simulink model "vehicle_directDrive_Torque"  (R2015a)
settings: Solver=ode23t  StartTime=0.0  StopTime=100  RelTol=1e-3  AbsTol=1e-3
PreLoadFcn:
  | car_tire_data
values from neighbouring files (symbols this model uses):
  rider_mass = 80    [car_tire_data.m]
  tire_dia = 18    [car_tire_data.m]
  vehicle_mass = 237    [car_tire_data.m]
libraries: fl_lib x13, nesl_utility x13, sdl_lib x5
settings Model: Creator=sseshadr  LastModifiedBy=sseshadr
settings SimscapeCC: SimscapeLogType=all  SimscapeLogDataHistory=10000

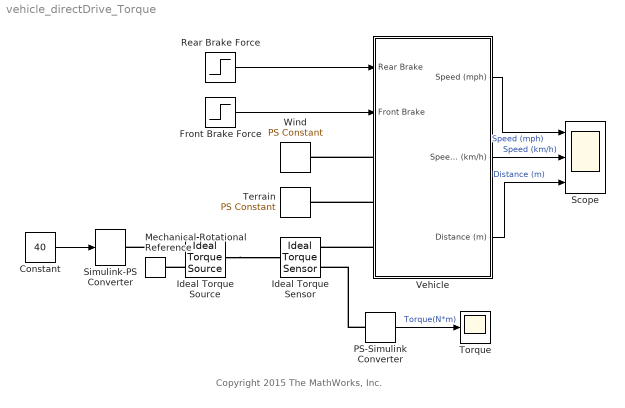
== system vehicle_directDrive_Torque ==
  note: Copyright 2015 The MathWorks, Inc.
  Constant : Constant  Value=40
  Front Brake Force : Step  Time=75  After=200  SampleTime=0
      settings: AttributesFormatString=%<After> N at %<Time> s
  Ideal Torque Sensor : fl_lib/Mechanical/Mechanical Sensors/Ideal Torque Sensor
  Ideal Torque Source : fl_lib/Mechanical/Mechanical Sources/Ideal Torque Source
  Mechanical Rotational Reference : fl_lib/Mechanical/Rotational Elements/Mechanical Rotational Reference
  PS-Simulink Converter : nesl_utility/PS-Simulink Converter  PhysicalDomain=network_engine_domain  SubClassName=ps_output  LeftPortType=input  RightPortType=output  PseudoPeriodic=off  Frequencies=[]  Unit=N*m  AffineConversion=off
  Rear Brake Force : Step  Time=50  After=100  SampleTime=0
      settings: AttributesFormatString=%<After> N at %<Time> s
  Scope : Scope  NumInputPorts=3
      settings: YMin=-5~-5~-5  YMax=5~5~5
  Simulink-PS Converter : nesl_utility/Simulink-PS Converter  PhysicalDomain=network_engine_domain  SubClassName=ps_input  LeftPortType=input  RightPortType=output  PseudoPeriodic=off  Frequencies=[]  NoiseDistribution=none  NoiseParameters=[]  Unit=N*m  AffineConversion=off  InputFiltering=off  SimscapeFilterOrder=1  InputFilterTimeConstant=0.001  UdotUserProvided=1
  Terrain : fl_lib/Physical Signals/Sources/PS Constant  constant=0
  Torque : Scope
      settings: TimeRange=40  YMin=-100  YMax=1000  SaveName=ScopeData2
  Vehicle : Subsystem
  Wind : fl_lib/Physical Signals/Sources/PS Constant  constant=0
  wires:
  Rear Brake Force/1 -> Vehicle/1(Rear Brake)
  Vehicle/1(Speed (mph)) -> Scope/1  "Speed (mph)"
  Vehicle/2(Speed (km/h)) -> Scope/2  "Speed (km/h)"
  Vehicle/3(Distance (m)) -> Scope/3  "Distance (m)"
  Front Brake Force/1 -> Vehicle/2(Front Brake)
  Constant/1 -> Simulink-PS Converter/1
  PS-Simulink Converter/1 -> Torque/1  "Torque(N*m)"
  connections:
  Vehicle/LConn1 -- Wind/RConn1
  Vehicle/LConn2 -- Terrain/RConn1
  Ideal Torque Source/RConn1 -- Simulink-PS Converter/RConn1
  Vehicle/LConn3 -- Ideal Torque Sensor/RConn1
  Ideal Torque Source/RConn2 -- Mechanical Rotational Reference/LConn1
  PS-Simulink Converter/LConn1 -- Ideal Torque Sensor/RConn2
  Ideal Torque Source/LConn1 -- Ideal Torque Sensor/LConn1

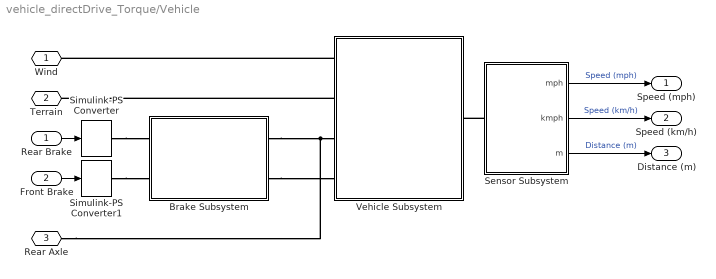
== system vehicle_directDrive_Torque/Vehicle ==
  Rear Brake : Inport
  Front Brake : Inport  Port=2
  Brake Subsystem : Subsystem
  Sensor Subsystem : Subsystem
  Simulink-PS Converter : nesl_utility/Simulink-PS Converter  PhysicalDomain=network_engine_domain  SubClassName=ps_input  LeftPortType=input  RightPortType=output  PseudoPeriodic=off  Frequencies=[]  NoiseDistribution=none  NoiseParameters=[]  Unit=1  AffineConversion=off  InputFiltering=on  SimscapeFilterOrder=1  InputFilterTimeConstant=0.001  UdotUserProvided=1
  Simulink-PS Converter1 : nesl_utility/Simulink-PS Converter  PhysicalDomain=network_engine_domain  SubClassName=ps_input  LeftPortType=input  RightPortType=output  PseudoPeriodic=off  Frequencies=[]  NoiseDistribution=none  NoiseParameters=[]  Unit=1  AffineConversion=off  InputFiltering=on  SimscapeFilterOrder=1  InputFilterTimeConstant=0.001  UdotUserProvided=1
  Vehicle Subsystem : Subsystem
  Wind : PMIOPort  Port=1  Side=Left
  Terrain : PMIOPort  Port=2  Side=Left
  Rear Axle : PMIOPort  Port=3  Side=Left
  Speed (mph) : Outport
  Speed (km/h) : Outport  Port=2
  Distance (m) : Outport  Port=3
  wires:
  Sensor Subsystem/1(mph) -> Speed (mph)/1  "Speed (mph)"
  Sensor Subsystem/2(kmph) -> Speed (km/h)/1  "Speed (km/h)"
  Sensor Subsystem/3(m) -> Distance (m)/1  "Distance (m)"
  Rear Brake/1 -> Simulink-PS Converter/1
  Front Brake/1 -> Simulink-PS Converter1/1
  connections:
  Simulink-PS Converter/RConn1 -- Brake Subsystem/LConn1
  Brake Subsystem/RConn1 -- Rear Axle/RConn1 -- Vehicle Subsystem/LConn3
  Brake Subsystem/RConn2 -- Vehicle Subsystem/LConn4
  Simulink-PS Converter1/RConn1 -- Brake Subsystem/LConn2
  Sensor Subsystem/LConn1 -- Vehicle Subsystem/RConn1
  Vehicle Subsystem/LConn1 -- Wind/RConn1
  Vehicle Subsystem/LConn2 -- Terrain/RConn1

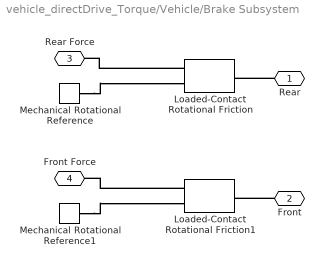
== system vehicle_directDrive_Torque/Vehicle/Brake Subsystem ==
  Loaded-Contact Rotational Friction : sdl_lib/Brakes & Detents/Rotational/Loaded-Contact Rotational Friction  geometry_model=1  r_eff=280 mm  d_o=150 mm  d_i=100 mm  friction_model=1  mu_coulomb=0.3  mu_w_vector=[ 0 0.1 0.2 0.3 0.4 0.5 1 2 5 10 100 1000 ] rad/s  mu_coulomb_vector=[ 0.29 0.28 0.26 0.22 0.21 0.2 0.2 0.19 0.19 0.19 0.19 0.19 ]  mu_interp_method=1  mu_extrap_method=1  mu_static=0.35  w_tol=0.001 rad/s  force_min=1 N  mu_visc=0 N*m/(rad/s)  initial_state_locked=0
  Loaded-Contact Rotational Friction1 : sdl_lib/Brakes & Detents/Rotational/Loaded-Contact Rotational Friction  geometry_model=1  r_eff=280 mm  d_o=150 mm  d_i=100 mm  friction_model=1  mu_coulomb=0.3  mu_w_vector=[ 0 0.1 0.2 0.3 0.4 0.5 1 2 5 10 100 1000 ] rad/s  mu_coulomb_vector=[ 0.29 0.28 0.26 0.22 0.21 0.2 0.2 0.19 0.19 0.19 0.19 0.19 ]  mu_interp_method=1  mu_extrap_method=1  mu_static=0.35  w_tol=0.001 rad/s  force_min=1 N  mu_visc=0 N*m/(rad/s)  initial_state_locked=0
  Mechanical Rotational Reference : fl_lib/Mechanical/Rotational Elements/Mechanical Rotational Reference
  Mechanical Rotational Reference1 : fl_lib/Mechanical/Rotational Elements/Mechanical Rotational Reference
  Rear : PMIOPort  Port=1  Side=Right
  Front : PMIOPort  Port=2  Side=Right
  Rear Force : PMIOPort  Port=3  Side=Left
  Front Force : PMIOPort  Port=4  Side=Left
  connections:
  Mechanical Rotational Reference/LConn1 -- Loaded-Contact Rotational Friction/LConn2
  Mechanical Rotational Reference1/LConn1 -- Loaded-Contact Rotational Friction1/LConn2
  Loaded-Contact Rotational Friction/LConn1 -- Rear Force/RConn1
  Loaded-Contact Rotational Friction1/LConn1 -- Front Force/RConn1
  Rear/RConn1 -- Loaded-Contact Rotational Friction/RConn1
  Front/RConn1 -- Loaded-Contact Rotational Friction1/RConn1

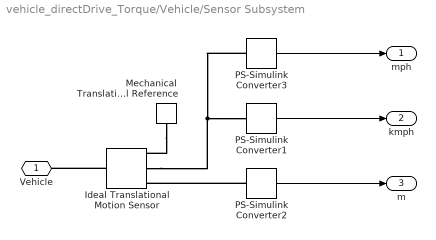
== system vehicle_directDrive_Torque/Vehicle/Sensor Subsystem ==
  Ideal Translational Motion Sensor : fl_lib/Mechanical/Mechanical Sensors/Ideal Translational Motion Sensor  offset=0 m
  Mechanical Translational Reference : fl_lib/Mechanical/Translational Elements/Mechanical Translational Reference
  PS-Simulink Converter1 : nesl_utility/PS-Simulink Converter  PhysicalDomain=network_engine_domain  SubClassName=ps_output  LeftPortType=input  RightPortType=output  PseudoPeriodic=off  Frequencies=[]  Unit=km/hr  AffineConversion=off
  PS-Simulink Converter2 : nesl_utility/PS-Simulink Converter  PhysicalDomain=network_engine_domain  SubClassName=ps_output  LeftPortType=input  RightPortType=output  PseudoPeriodic=off  Frequencies=[]  Unit=1  AffineConversion=off
  PS-Simulink Converter3 : nesl_utility/PS-Simulink Converter  PhysicalDomain=network_engine_domain  SubClassName=ps_output  LeftPortType=input  RightPortType=output  PseudoPeriodic=off  Frequencies=[]  Unit=mph  AffineConversion=off
  Vehicle : PMIOPort  Port=1  Side=Left
  mph : Outport
  kmph : Outport  Port=2
  m : Outport  Port=3
  wires:
  PS-Simulink Converter1/1 -> kmph/1
  PS-Simulink Converter2/1 -> m/1
  PS-Simulink Converter3/1 -> mph/1
  connections:
  Mechanical Translational Reference/LConn1 -- Ideal Translational Motion Sensor/RConn1
  PS-Simulink Converter2/LConn1 -- Ideal Translational Motion Sensor/RConn3
  Ideal Translational Motion Sensor/RConn2 -- PS-Simulink Converter3/LConn1 -- PS-Simulink Converter1/LConn1
  Ideal Translational Motion Sensor/LConn1 -- Vehicle/RConn1

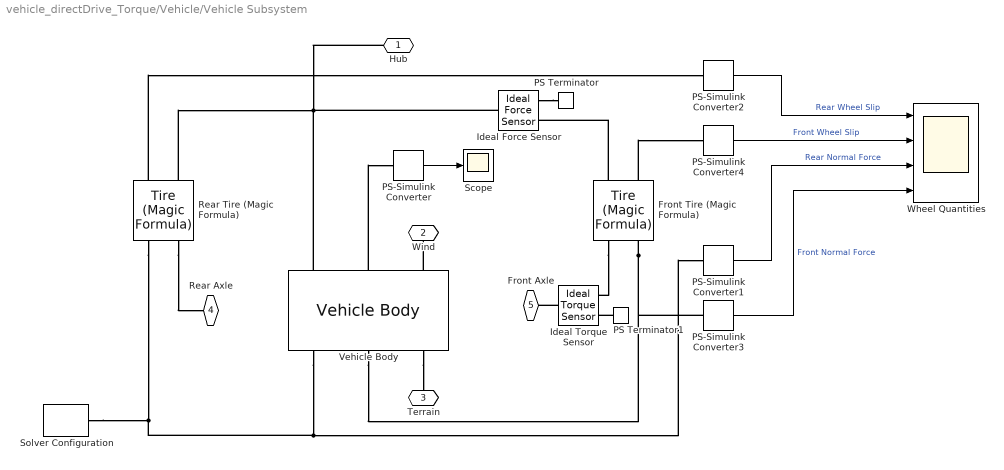
== system vehicle_directDrive_Torque/Vehicle/Vehicle Subsystem ==
  Front Tire (Magic Formula) : sdl_lib/Tires & Vehicles/Tire (Magic Formula)  parameterization=2  F_z1=3e+3 N  F_x1=3.5e+3 N  kappa1=10  B_m=tire_b  C_m=tire_c  D_m=tire_d  E_m=tire_e  fz0=4e+3 N  p_Cx=1.685  p_Dx=[ 1.21 -0.037 ]  p_Ex=[ 0.344 0.095 -0.02 0 ]  p_Kx=[ 21.51 -0.163 0.245 ]  p_Hx=[ -0.002 0.002 ]  p_Vx=[ 0 0 ]  v_tr_thr=0.1 m/s  r_e=tire_dia/2 in  model_compliance=0  stiffness=1e+6 N/m  damping=1000 N/(m/s)  model_inertia=1  inertia=tire_inertia kg*m^2  initial_velocity=0 rad/s  model_resistance=1  resistance_model=1  coeff=roll_resist  p_tire=250e3 Pa  alpha=-0.003  beta=0.97  coeff_a=84e-4  coeff_b=6.2e-4 s/m  coeff_c=1.6e-4 s^2/m^2  v_thr=1e-3 m/s
  Ideal Force Sensor : fl_lib/Mechanical/Mechanical Sensors/Ideal Force Sensor
  Ideal Torque Sensor : fl_lib/Mechanical/Mechanical Sensors/Ideal Torque Sensor
  PS Terminator : fl_lib/Physical Signals/Sinks/PS Terminator
  PS Terminator1 : fl_lib/Physical Signals/Sinks/PS Terminator
  PS-Simulink Converter : nesl_utility/PS-Simulink Converter  PhysicalDomain=network_engine_domain  SubClassName=ps_output  LeftPortType=input  RightPortType=output  PseudoPeriodic=off  Frequencies=[]  Unit=1  AffineConversion=off
  PS-Simulink Converter{1..4} (4 alike) : nesl_utility/PS-Simulink Converter  PhysicalDomain=network_engine_domain  SubClassName=ps_output  LeftPortType=input  RightPortType=output  PseudoPeriodic=off  Frequencies=[]  Unit=N  AffineConversion=off
  Rear Tire (Magic Formula) : sdl_lib/Tires & Vehicles/Tire (Magic Formula)  parameterization=2  F_z1=3e+3 N  F_x1=3.5e+3 N  kappa1=10  B_m=tire_b  C_m=tire_c  D_m=tire_d  E_m=tire_e  fz0=4e+3 N  p_Cx=1.685  p_Dx=[ 1.21 -0.037 ]  p_Ex=[ 0.344 0.095 -0.02 0 ]  p_Kx=[ 21.51 -0.163 0.245 ]  p_Hx=[ -0.002 0.002 ]  p_Vx=[ 0 0 ]  v_tr_thr=0.1 m/s  r_e=tire_dia/2 in  model_compliance=0  stiffness=1e+6 N/m  damping=1000 N/(m/s)  model_inertia=1  inertia=tire_inertia kg*m^2  initial_velocity=0 rad/s  model_resistance=1  resistance_model=1  coeff=roll_resist  p_tire=250e3 Pa  alpha=-0.003  beta=0.97  coeff_a=84e-4  coeff_b=6.2e-4 s/m  coeff_c=1.6e-4 s^2/m^2  v_thr=1e-3 m/s
  Scope : Scope
  Solver Configuration : nesl_utility/Solver Configuration  PhysicalDomain=network_engine_domain  SubClassName=solver  LeftPortType=input  RightPortType=generic  Accelerate=off  Tones=[]  Harmonics=[]  SimulateNoise=off  Profile=off  UseLocalSampling=off  EnableSwitchedLinearOptims=on  FrequencyDomain=off  UseCCode=off  RelTol=0.001  AbsTol=1e-06  MinStep=1e-09  ToWorkspace=off  RevertToSquareIcSolve=off  NumHomotopyIterations=100  DoDC=off  ResidualTolerance=1e-09  UseLocalSolver=off  LocalSolverChoice=NE_BACKWARD_EULER_ADVANCER  LocalSolverSampleTime=0.001  DoFixedCost=off  MaxNonlinIter=3  MaxModeIter=2  LinearAlgebra=Sparse  DelaysMemoryBudget=1024  AutomaticFiltering=on  FilteringTimeConstant=0.001
  Vehicle Body : sdl_lib/Tires & Vehicles/Vehicle Body  mass=rider_mass + vehicle_mass kg  n_w=1  x_f=front_axle mm  x_r=rear_axle mm  y_c=CG_height mm  area=front_area m^2  Cd=drag_coeff  v0=0 m/s  g=9.81 m/s^2  rho=1.18 kg/m^3
  Wheel Quantities : Scope  NumInputPorts=4
      settings: TimeRange=75  YMin=-1.739899074664905~-0.00106484112383577~1490.505319148936~-500.1976734211385  YMax=46.19404070580568~0.0003082650279803026~1497.845744680851~48.06634367574588  SaveName=ScopeData3
  Hub : PMIOPort  Port=1  Side=Right
  Wind : PMIOPort  Port=2  Side=Left
  Terrain : PMIOPort  Port=3  Side=Left
  Rear Axle : PMIOPort  Port=4  Side=Left
  Front Axle : PMIOPort  Port=5  Side=Left
  wires:
  PS-Simulink Converter/1 -> Scope/1
  PS-Simulink Converter2/1 -> Wheel Quantities/1  "Rear Wheel Slip"
  PS-Simulink Converter4/1 -> Wheel Quantities/2  "Front Wheel Slip"
  PS-Simulink Converter1/1 -> Wheel Quantities/3  "Rear Normal Force"
  PS-Simulink Converter3/1 -> Wheel Quantities/4  "Front Normal Force"
  connections:
  Vehicle Body/RConn1 -- Solver Configuration/RConn1 -- Rear Tire (Magic Formula)/LConn1 -- PS-Simulink Converter1/LConn1
  Front Tire (Magic Formula)/LConn1 -- Vehicle Body/RConn2 -- PS-Simulink Converter3/LConn1
  Vehicle Body/LConn2 -- PS-Simulink Converter/LConn1
  Ideal Force Sensor/LConn1 -- Rear Tire (Magic Formula)/RConn2 -- Vehicle Body/LConn1 -- Hub/RConn1
  Vehicle Body/LConn3 -- Wind/RConn1
  Vehicle Body/RConn3 -- Terrain/RConn1
  Rear Tire (Magic Formula)/LConn2 -- Rear Axle/RConn1
  Front Tire (Magic Formula)/RConn2 -- Ideal Force Sensor/RConn1
  Ideal Torque Sensor/LConn1 -- Front Axle/RConn1
  Front Tire (Magic Formula)/LConn2 -- Ideal Torque Sensor/RConn1
  Front Tire (Magic Formula)/RConn1 -- PS-Simulink Converter4/LConn1
  Rear Tire (Magic Formula)/RConn1 -- PS-Simulink Converter2/LConn1
  Ideal Force Sensor/RConn2 -- PS Terminator/LConn1
  PS Terminator1/LConn1 -- Ideal Torque Sensor/RConn2
